simulink model "control_system"  (R2015a)
settings: Solver=ode45  StartTime=0.0  StopTime=36e4  RelTol=1e-3
values from neighbouring files (symbols this model uses):
  StepDist = 0    [Main.m]
  StepTime = 1200    [Main.m]
settings Model: CovSFcnEnable=off  Creator=Piotr  LastModifiedBy=Piotr
settings DebuggingCC: UnderspecifiedInitializationDetection=Classic  MergeDetectMultiDrivingBlocksExec=none  SolverPrmCheckMsg=warning  StateNameClashWarn=warning

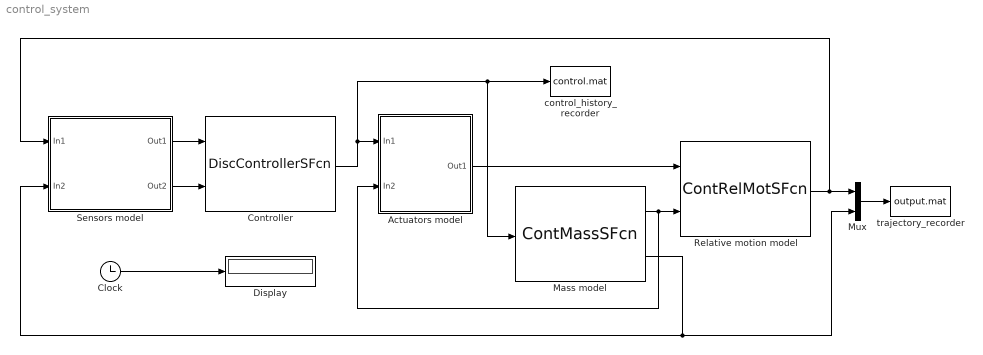
== system control_system ==
  Actuators model : Subsystem
  Clock : Clock
  Controller : M-S-Function  FunctionName=DiscControllerSFcn  Parameters=SimulationScenario
  Display : Display
  Mass model : M-S-Function  FunctionName=ContMassSFcn  Parameters=SimulationScenario
  Mux : Mux  Inputs=2
  Relative motion model : M-S-Function  FunctionName=ContRelMotSFcn  Parameters=SimulationScenario
  Sensors model : Subsystem
  control_history_recorder : ToFile  Filename=control.mat  MatrixName=ControlHistory  SaveFormat=Timeseries  SampleTime=300
      settings: AttributesFormatString=%<SampleTime>
  trajectory_recorder : ToFile  Filename=output.mat  MatrixName=OutputHistory  SaveFormat=Timeseries  SampleTime=300
      settings: AttributesFormatString=%<SampleTime>
  wires:
  Actuators model/1(Out1) -> Relative motion model/1
  Mass model/1 -> Actuators model/2(In2), Relative motion model/2
  Relative motion model/1 -> Sensors model/1(In1), Mux/1
  Clock/1 -> Display/1
  Mass model/2 -> Sensors model/2(In2), Mux/2
  Mux/1 -> trajectory_recorder/1
  Sensors model/1(Out1) -> Controller/1
  Sensors model/2(Out2) -> Controller/2
  Controller/1 -> Mass model/1, control_history_recorder/1, Actuators model/1(In1)

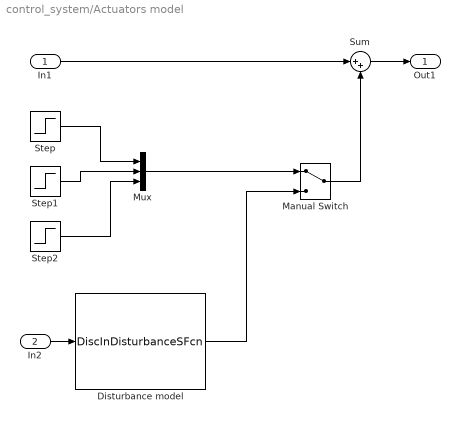
== system control_system/Actuators model ==
  In1 : Inport
  In2 : Inport  Port=2
  Disturbance model : M-S-Function  FunctionName=DiscInDisturbanceSFcn  Parameters=SimulationScenario
  Manual Switch : ManualSwitch
  Mux : Mux  Inputs=3
  Step : Step  Time=StepTime  After=StepDist  SampleTime=0
  Step1 : Step  Time=StepTime  After=StepDist  SampleTime=0
  Step2 : Step  Time=StepTime  After=StepDist  SampleTime=0
  Sum : Sum  Inputs=|++
  Out1 : Outport
  wires:
  In1/1 -> Sum/1
  Sum/1 -> Out1/1
  In2/1 -> Disturbance model/1
  Manual Switch/1 -> Sum/2
  Disturbance model/1 -> Manual Switch/2
  Step/1 -> Mux/1
  Step1/1 -> Mux/2
  Step2/1 -> Mux/3
  Mux/1 -> Manual Switch/1

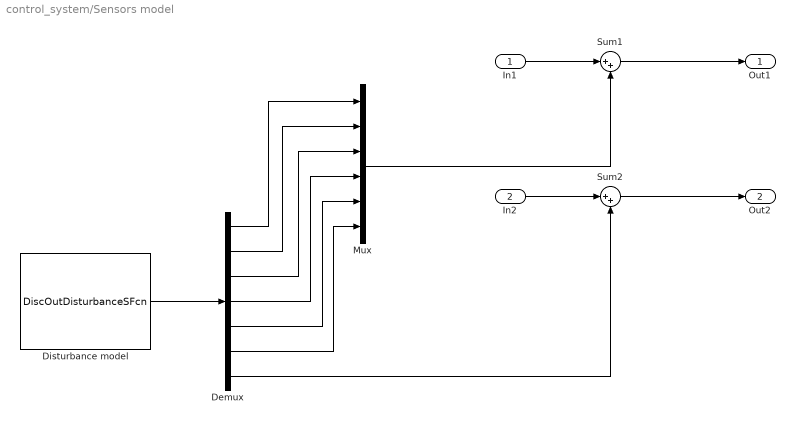
== system control_system/Sensors model ==
  In1 : Inport
  In2 : Inport  Port=2
  Demux : Demux  Outputs=7
  Disturbance model : M-S-Function  FunctionName=DiscOutDisturbanceSFcn  Parameters=SimulationScenario
  Mux : Mux  Inputs=6
  Sum1 : Sum  Inputs=|++
  Sum2 : Sum  Inputs=|++
  Out1 : Outport
  Out2 : Outport  Port=2
  wires:
  In1/1 -> Sum1/1
  Sum1/1 -> Out1/1
  In2/1 -> Sum2/1
  Sum2/1 -> Out2/1
  Disturbance model/1 -> Demux/1
  Demux/6 -> Mux/6
  Demux/5 -> Mux/5
  Demux/4 -> Mux/4
  Demux/3 -> Mux/3
  Demux/2 -> Mux/2
  Demux/1 -> Mux/1
  Mux/1 -> Sum1/2
  Demux/7 -> Sum2/2
